simulink model "ss_lin_sys"  (R2020a)
settings: Solver=VariableStepAuto  StartTime=0.0  StopTime=300  RelTol=1e-9
undefined symbols (not defined in the file): a, A, B, C, D, IC_lin, omega
settings Model: Creator=Tomo  LastModifiedBy=Tomo

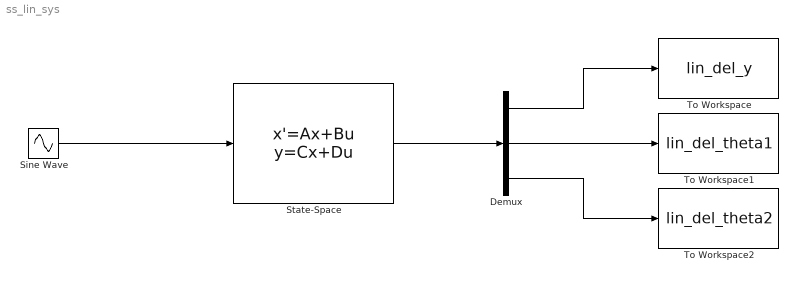
== system ss_lin_sys ==
  Demux : Demux  Outputs=3
  Sine Wave : Sin  Amplitude=a  Frequency=omega  SampleTime=0
  State-Space : StateSpace  A=A  B=B  C=C  D=D  InitialCondition=IC_lin
  To Workspace : ToWorkspace  VariableName=lin_del_y  SaveFormat=Structure With Time  SampleTime=-1
  To Workspace1 : ToWorkspace  VariableName=lin_del_theta1  SaveFormat=Structure With Time  SampleTime=-1
  To Workspace2 : ToWorkspace  VariableName=lin_del_theta2  SaveFormat=Structure With Time  SampleTime=-1
  wires:
  Sine Wave/1 -> State-Space/1
  State-Space/1 -> Demux/1
  Demux/1 -> To Workspace/1
  Demux/2 -> To Workspace1/1
  Demux/3 -> To Workspace2/1
